simulink library "csc_lpr_lidar_short_long_range_pair_lib"  (R2015b)
settings: Solver=ode45  SolverMode=SingleTasking  StartTime=0.0  StopTime=10.0  RelTol=1e-3
undefined symbols (not defined in the file): lander_dcm, ldr1_lander_dcm, ldr1_lander_pos, position_in_lander
libraries: csu_flr_lidar_noise_model_lib x4, csu_rng_range_model_lib x4, util_common_lib x4, util_info_lib x2
settings Model: Creator=eleanor  LastModifiedBy=Mark Agbayani
settings DataIOCC: SaveFormat=Array  SignalLoggingSaveFormat=ModelDataLogs
settings OptimizationCC: BlockReduction=off  BooleanDataType=off  ExpressionDepthLimit=2147483647
settings DebuggingCC: SaveWithParameterizedLinksMsg=none  UnderspecifiedInitializationDetection=Classic  MergeDetectMultiDrivingBlocksExec=none  SignalResolutionControl=TryResolveAllWithWarning  FcnCallInpInsideContextMsg=EnableAllAsWarning  StateNameClashWarn=warning  StrictBusMsg=Warning
settings HardwareCC: ProdBitPerPointer=32  ProdLargestAtomicFloat=None  ProdIntDivRoundTo=Undefined  ProdEndianess=Unspecified  ProdWordSize=32  ProdHWDeviceType=32-bit Generic  TargetUnknown=on
settings GRTTargetCC: GeneratePreprocessorConditionals=Disable all  CombineOutputUpdateFcns=off  GRTInterface=on
settings ConfigComp: CovModelRefEnable=Off  CovSFcnEnable=off

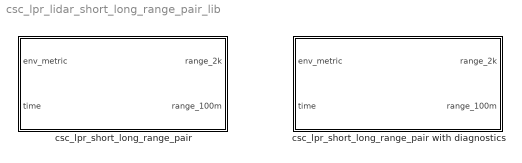
== system csc_lpr_lidar_short_long_range_pair_lib ==
  csc_lpr_short_long_range_pair : Subsystem  SystemSampleTime=0.1  mask{position_in_lander=position_in_lander, lander_dcm=lander_dcm}
      mask prompts: position_in_lander "LIDAR Position in Body Frame (meters)"; lander_dcm "LIDAR Attitude wrt Body Frame (DCM)"
  csc_lpr_short_long_range_pair with diagnostics : Subsystem  AncestorBlock=csc_lpr_lidar_short_long_range_pair_lib/csc_lpr_short_long_range_pair  SystemSampleTime=0.1  mask{position_in_lander=ldr1_lander_pos, lander_dcm=ldr1_lander_dcm}
      mask prompts: position_in_lander "LIDAR Position in Body Frame (meters)"; lander_dcm "LIDAR Attitude wrt Body Frame (DCM)"

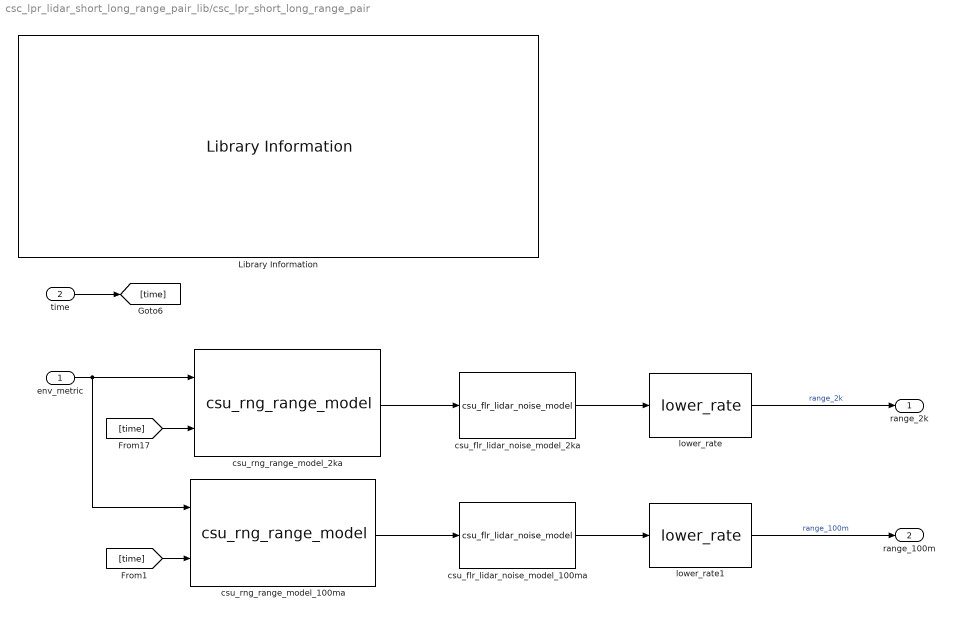
== system csc_lpr_lidar_short_long_range_pair_lib/csc_lpr_short_long_range_pair ==
  env_metric : Inport
  time : Inport  Port=2
  Library Information : util_info_lib/Library Information  owner='escrane'
  csu_flr_lidar_noise_model_100ma : csu_flr_lidar_noise_model_lib/csu_flr_lidar_noise_model  model_type=flr_100m_model
  csu_flr_lidar_noise_model_2ka : csu_flr_lidar_noise_model_lib/csu_flr_lidar_noise_model  model_type=flr_2k_model
  csu_rng_range_model_100ma : csu_rng_range_model_lib/csu_rng_range_model  position_in_lander=position_in_lander  lander_dcm=lander_dcm
  csu_rng_range_model_2ka : csu_rng_range_model_lib/csu_rng_range_model  position_in_lander=position_in_lander  lander_dcm=lander_dcm
  lower_rate : util_common_lib/lower_rate  counter_max=flr_2k_rate_counter  counter_init=0
  lower_rate1 : util_common_lib/lower_rate  counter_max=flr_100m_rate_counter  counter_init=0
  range_2k : Outport
  range_100m : Outport  Port=2
  wires:
  [time] -> csu_rng_range_model_100ma/2
  time/1 -> [time]
  [time] -> csu_rng_range_model_2ka/2
  lower_rate1/1 -> range_100m/1  "range_100m"
  csu_rng_range_model_100ma/1 -> csu_flr_lidar_noise_model_100ma/1
  csu_flr_lidar_noise_model_100ma/1 -> lower_rate1/1
  env_metric/1 -> csu_rng_range_model_2ka/1, csu_rng_range_model_100ma/1
  lower_rate/1 -> range_2k/1  "range_2k"
  csu_rng_range_model_2ka/1 -> csu_flr_lidar_noise_model_2ka/1
  csu_flr_lidar_noise_model_2ka/1 -> lower_rate/1

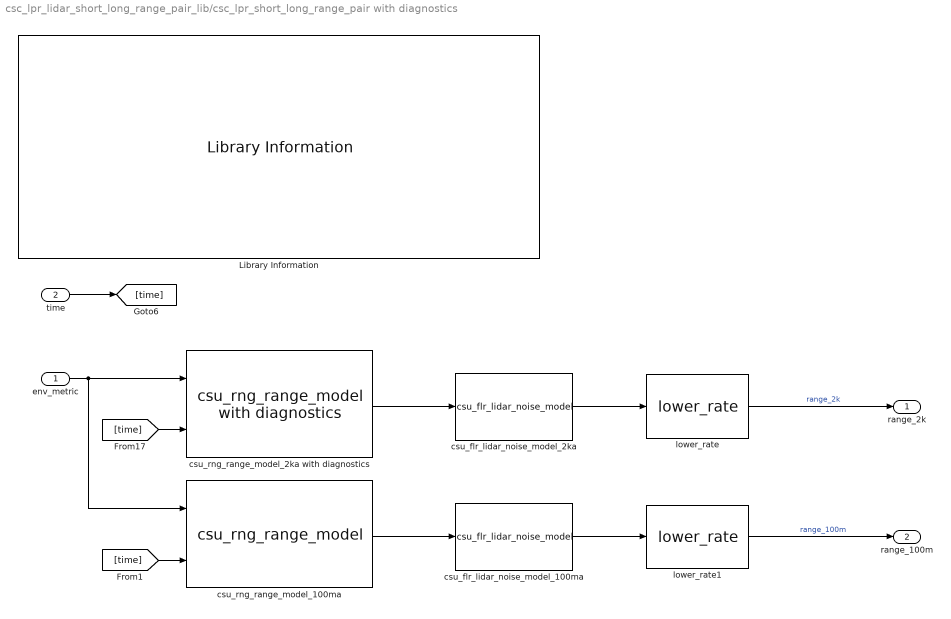
== system csc_lpr_lidar_short_long_range_pair_lib/csc_lpr_short_long_range_pair with diagnostics ==
  env_metric : Inport
  time : Inport  Port=2
  Library Information : util_info_lib/Library Information  owner='escrane'
  csu_flr_lidar_noise_model_100ma : csu_flr_lidar_noise_model_lib/csu_flr_lidar_noise_model  model_type=flr_100m_model
  csu_flr_lidar_noise_model_2ka : csu_flr_lidar_noise_model_lib/csu_flr_lidar_noise_model  model_type=flr_2k_model
  csu_rng_range_model_100ma : csu_rng_range_model_lib/csu_rng_range_model  position_in_lander=position_in_lander  lander_dcm=lander_dcm
  csu_rng_range_model_2ka with diagnostics : csu_rng_range_model_lib/csu_rng_range_model with diagnostics  position_in_lander=position_in_lander  lander_dcm=lander_dcm
  lower_rate : util_common_lib/lower_rate  counter_max=flr_2k_rate_counter  counter_init=0
  lower_rate1 : util_common_lib/lower_rate  counter_max=flr_100m_rate_counter  counter_init=0
  range_2k : Outport
  range_100m : Outport  Port=2
  wires:
  csu_flr_lidar_noise_model_2ka/1 -> lower_rate/1
  csu_rng_range_model_2ka with diagnostics/1 -> csu_flr_lidar_noise_model_2ka/1
  lower_rate/1 -> range_2k/1  "range_2k"
  env_metric/1 -> csu_rng_range_model_2ka with diagnostics/1, csu_rng_range_model_100ma/1
  csu_flr_lidar_noise_model_100ma/1 -> lower_rate1/1
  csu_rng_range_model_100ma/1 -> csu_flr_lidar_noise_model_100ma/1
  lower_rate1/1 -> range_100m/1  "range_100m"
  [time] -> csu_rng_range_model_2ka with diagnostics/2
  time/1 -> [time]
  [time] -> csu_rng_range_model_100ma/2
